simulink model "Demo_V2X_RoadWorks_cs"  (R2014b)
settings: Solver=ode5  SolverMode=SingleTasking  StartTime=0.0  StopTime=18  FixedStep=1/100  RelTol=1e-3
PreLoadFcn:
  | mbxruntime.callbacks.PreLoadFcn(bdroot);
  | check_NUTS_defined;
  | 
  | assignin('base',['model_closed_' bdroot],false);
PostLoadFcn:
  | mbxruntime.callbacks.PostLoadFcn(bdroot);
InitFcn:
  | mbxruntime.callbacks.InitFcn(bdroot);
StartFcn:
  | mbxruntime.callbacks.StartFcn(bdroot);
StopFcn:
  | mbxruntime.callbacks.StopFcn(bdroot);
model workspace: external: MAT-File .\Demo_V2X_RoadWorks_cs_hws.mat (data not in the file)
undefined symbols (not defined in the file or in its folder): InitializeBus, mbxruntime, Newton, Raphson, tabledata
undefined symbols (not defined in the file): Demo_V2X_RoadWorks_cs_002408181c311178, Demo_V2X_RoadWorks_cs_02afd40c5576fd79, Demo_V2X_RoadWorks_cs_09062d95c4976b80, Demo_V2X_RoadWorks_cs_0ad60e46608f1bfe, Demo_V2X_RoadWorks_cs_0b386a01b2cd5e8d, Demo_V2X_RoadWorks_cs_0d795afaa024d2ee, Demo_V2X_RoadWorks_cs_104085e65c337077, Demo_V2X_RoadWorks_cs_126564f7b2997a49, Demo_V2X_RoadWorks_cs_15e6e2595e8bf329, Demo_V2X_RoadWorks_cs_16adfea7655bce18, Demo_V2X_RoadWorks_cs_18ab2686f8449f50, Demo_V2X_RoadWorks_cs_1c28437def32f9f6, Demo_V2X_RoadWorks_cs_1d541c73c3d8f25b, Demo_V2X_RoadWorks_cs_1fb1f994fe012d27, Demo_V2X_RoadWorks_cs_20c117b9827230b9, Demo_V2X_RoadWorks_cs_220b1226a84e3b37, Demo_V2X_RoadWorks_cs_24814049c8ab2e18, Demo_V2X_RoadWorks_cs_24a281220a6492a7, Demo_V2X_RoadWorks_cs_279aea126b4236ad, Demo_V2X_RoadWorks_cs_28eadd0b23e572db, Demo_V2X_RoadWorks_cs_291fe7210f9ba434, Demo_V2X_RoadWorks_cs_2fd90504f8814746, Demo_V2X_RoadWorks_cs_33c1737bfc1c651f, Demo_V2X_RoadWorks_cs_388e22d5b1056b8f, Demo_V2X_RoadWorks_cs_3e3a415e868663e7, Demo_V2X_RoadWorks_cs_45759eb0c1816b1e, Demo_V2X_RoadWorks_cs_45f301cf6c396570, Demo_V2X_RoadWorks_cs_47686124f5151dea, Demo_V2X_RoadWorks_cs_487931e8a8cef1d6, Demo_V2X_RoadWorks_cs_54cb5626dca53ab7, Demo_V2X_RoadWorks_cs_56c0a253fe7e7ec0, Demo_V2X_RoadWorks_cs_5921488c0ba4168e, Demo_V2X_RoadWorks_cs_5ca0c70551eea1b3, Demo_V2X_RoadWorks_cs_5cc6ddb60eb17926, Demo_V2X_RoadWorks_cs_5dda33a127b53dd9, Demo_V2X_RoadWorks_cs_60729aca19e3b8ea, Demo_V2X_RoadWorks_cs_61616eaaf58ec115, Demo_V2X_RoadWorks_cs_63af626c9fae5224, Demo_V2X_RoadWorks_cs_649c6af7b111a61f, Demo_V2X_RoadWorks_cs_64e2df335ac415c1, Demo_V2X_RoadWorks_cs_6530f1ae727e39fe, Demo_V2X_RoadWorks_cs_6837be8d052ff1e3, Demo_V2X_RoadWorks_cs_6e8b51a123f1a201, Demo_V2X_RoadWorks_cs_6f4ec518a68cacb3, Demo_V2X_RoadWorks_cs_74dac4a6b9859226, Demo_V2X_RoadWorks_cs_75671d8cae67d5b6, Demo_V2X_RoadWorks_cs_756d40a88ae84d39, Demo_V2X_RoadWorks_cs_77c7cbc4fa1cdaa5, Demo_V2X_RoadWorks_cs_7b9fbc44403bb8f3, Demo_V2X_RoadWorks_cs_7c118b74c8d14c00, Demo_V2X_RoadWorks_cs_7c4a172761f05beb, Demo_V2X_RoadWorks_cs_80b7a78efe24d5f1, Demo_V2X_RoadWorks_cs_82d65efce1f7c4ea, Demo_V2X_RoadWorks_cs_8be5dc2565229ce9, Demo_V2X_RoadWorks_cs_8dc36f0ab6cec640, Demo_V2X_RoadWorks_cs_91305dd1362bb00d, Demo_V2X_RoadWorks_cs_929c2ffed1faf33f, Demo_V2X_RoadWorks_cs_95615bcbc0d062f1, Demo_V2X_RoadWorks_cs_99a6391a40f894df, Demo_V2X_RoadWorks_cs_9caa19175765ea5d ... (+52)
libraries: PreScanSimulinkLibrary x34, simulink_extras x15, simulink x6
(part 6 of 16)

== system Demo_V2X_RoadWorks_cs/V2X_Tx6196_DENM_Transmitter ==
  V2X_Tx6196_DENM_Transmitter : Inport  Tag=inport/plugin/sfun_V2X_DENM_Transmitter  BusOutputAsStruct=on
  Actuator : S-Function  FunctionName=sfun_V2X_DENM_Transmitter  Parameters=sensorID, parentID, timestep  EnableBusSupport=off  mask(V2X DENM Transmitter Block){sensorID=6196, parentID=3534, timestep=1/100}
      mask prompts: sensorID "Transmitter ID"; parentID "Parent ID"; timestep "MATLAB timestep:"
      mask help: V2X Block transmitting a DENM message
      mask Display: image(imread('V2XT_grayscale.png'))
  wires:
  V2X_Tx6196_DENM_Transmitter/1 -> Actuator/1

== system Demo_V2X_RoadWorks_cs/V2X_Tx6197_CAM_Transmitter ==
  V2X_Tx6197_CAM_Transmitter : Inport  Tag=inport/plugin/sfun_V2X_CAM_Transmitter  BusOutputAsStruct=on
  Actuator : S-Function  FunctionName=sfun_V2X_CAM_Transmitter  Parameters=sensorID, parentID, timestep  EnableBusSupport=off  mask(V2X CAM Transmitter Block){sensorID=6197, parentID=3535, timestep=1/100}
      mask prompts: sensorID "Transmitter ID"; parentID "Parent ID"; timestep "MATLAB timestep:"
      mask help: V2X Block transmitting a CAM message
      mask Display: image(imread('V2XT_grayscale.png'))
  wires:
  V2X_Tx6197_CAM_Transmitter/1 -> Actuator/1

== system Demo_V2X_RoadWorks_cs/V2X_Tx6197_DENM_Transmitter ==
  V2X_Tx6197_DENM_Transmitter : Inport  Tag=inport/plugin/sfun_V2X_DENM_Transmitter  BusOutputAsStruct=on
  Actuator : S-Function  FunctionName=sfun_V2X_DENM_Transmitter  Parameters=sensorID, parentID, timestep  EnableBusSupport=off  mask(V2X DENM Transmitter Block){sensorID=6197, parentID=3535, timestep=1/100}
      mask prompts: sensorID "Transmitter ID"; parentID "Parent ID"; timestep "MATLAB timestep:"
      mask help: V2X Block transmitting a DENM message
      mask Display: image(imread('V2XT_grayscale.png'))
  wires:
  V2X_Tx6197_DENM_Transmitter/1 -> Actuator/1

== system Demo_V2X_RoadWorks_cs/V2X_Tx6198_CAM_Transmitter ==
  V2X_Tx6198_CAM_Transmitter : Inport  Tag=inport/plugin/sfun_V2X_CAM_Transmitter  BusOutputAsStruct=on
  Actuator : S-Function  FunctionName=sfun_V2X_CAM_Transmitter  Parameters=sensorID, parentID, timestep  EnableBusSupport=off  mask(V2X CAM Transmitter Block){sensorID=6198, parentID=3606, timestep=1/100}
      mask prompts: sensorID "Transmitter ID"; parentID "Parent ID"; timestep "MATLAB timestep:"
      mask help: V2X Block transmitting a CAM message
      mask Display: image(imread('V2XT_grayscale.png'))
  wires:
  V2X_Tx6198_CAM_Transmitter/1 -> Actuator/1

== system Demo_V2X_RoadWorks_cs/V2X_Tx6198_DENM_Transmitter ==
  V2X_Tx6198_DENM_Transmitter : Inport  Tag=inport/plugin/sfun_V2X_DENM_Transmitter  BusOutputAsStruct=on
  Actuator : S-Function  FunctionName=sfun_V2X_DENM_Transmitter  Parameters=sensorID, parentID, timestep  EnableBusSupport=off  mask(V2X DENM Transmitter Block){sensorID=6198, parentID=3606, timestep=1/100}
      mask prompts: sensorID "Transmitter ID"; parentID "Parent ID"; timestep "MATLAB timestep:"
      mask help: V2X Block transmitting a DENM message
      mask Display: image(imread('V2XT_grayscale.png'))
  wires:
  V2X_Tx6198_DENM_Transmitter/1 -> Actuator/1

== system Demo_V2X_RoadWorks_cs/V2X_Tx6199_CAM_Transmitter ==
  V2X_Tx6199_CAM_Transmitter : Inport  Tag=inport/plugin/sfun_V2X_CAM_Transmitter  BusOutputAsStruct=on
  Actuator : S-Function  FunctionName=sfun_V2X_CAM_Transmitter  Parameters=sensorID, parentID, timestep  EnableBusSupport=off  mask(V2X CAM Transmitter Block){sensorID=6199, parentID=3607, timestep=1/100}
      mask prompts: sensorID "Transmitter ID"; parentID "Parent ID"; timestep "MATLAB timestep:"
      mask help: V2X Block transmitting a CAM message
      mask Display: image(imread('V2XT_grayscale.png'))
  wires:
  V2X_Tx6199_CAM_Transmitter/1 -> Actuator/1

== system Demo_V2X_RoadWorks_cs/V2X_Tx6199_DENM_Transmitter ==
  V2X_Tx6199_DENM_Transmitter : Inport  Tag=inport/plugin/sfun_V2X_DENM_Transmitter  BusOutputAsStruct=on
  Actuator : S-Function  FunctionName=sfun_V2X_DENM_Transmitter  Parameters=sensorID, parentID, timestep  EnableBusSupport=off  mask(V2X DENM Transmitter Block){sensorID=6199, parentID=3607, timestep=1/100}
      mask prompts: sensorID "Transmitter ID"; parentID "Parent ID"; timestep "MATLAB timestep:"
      mask help: V2X Block transmitting a DENM message
      mask Display: image(imread('V2XT_grayscale.png'))
  wires:
  V2X_Tx6199_DENM_Transmitter/1 -> Actuator/1

== system Demo_V2X_RoadWorks_cs/V2X_Tx6200_CAM_Transmitter ==
  V2X_Tx6200_CAM_Transmitter : Inport  Tag=inport/plugin/sfun_V2X_CAM_Transmitter  BusOutputAsStruct=on
  Actuator : S-Function  FunctionName=sfun_V2X_CAM_Transmitter  Parameters=sensorID, parentID, timestep  EnableBusSupport=off  mask(V2X CAM Transmitter Block){sensorID=6200, parentID=3608, timestep=1/100}
      mask prompts: sensorID "Transmitter ID"; parentID "Parent ID"; timestep "MATLAB timestep:"
      mask help: V2X Block transmitting a CAM message
      mask Display: image(imread('V2XT_grayscale.png'))
  wires:
  V2X_Tx6200_CAM_Transmitter/1 -> Actuator/1

== system Demo_V2X_RoadWorks_cs/V2X_Tx6200_DENM_Transmitter ==
  V2X_Tx6200_DENM_Transmitter : Inport  Tag=inport/plugin/sfun_V2X_DENM_Transmitter  BusOutputAsStruct=on
  Actuator : S-Function  FunctionName=sfun_V2X_DENM_Transmitter  Parameters=sensorID, parentID, timestep  EnableBusSupport=off  mask(V2X DENM Transmitter Block){sensorID=6200, parentID=3608, timestep=1/100}
      mask prompts: sensorID "Transmitter ID"; parentID "Parent ID"; timestep "MATLAB timestep:"
      mask help: V2X Block transmitting a DENM message
      mask Display: image(imread('V2XT_grayscale.png'))
  wires:
  V2X_Tx6200_DENM_Transmitter/1 -> Actuator/1

== system Demo_V2X_RoadWorks_cs/V2X_Tx6201_CAM_Transmitter ==
  V2X_Tx6201_CAM_Transmitter : Inport  Tag=inport/plugin/sfun_V2X_CAM_Transmitter  BusOutputAsStruct=on
  Actuator : S-Function  FunctionName=sfun_V2X_CAM_Transmitter  Parameters=sensorID, parentID, timestep  EnableBusSupport=off  mask(V2X CAM Transmitter Block){sensorID=6201, parentID=3609, timestep=1/100}
      mask prompts: sensorID "Transmitter ID"; parentID "Parent ID"; timestep "MATLAB timestep:"
      mask help: V2X Block transmitting a CAM message
      mask Display: image(imread('V2XT_grayscale.png'))
  wires:
  V2X_Tx6201_CAM_Transmitter/1 -> Actuator/1

== system Demo_V2X_RoadWorks_cs/V2X_Tx6201_DENM_Transmitter ==
  V2X_Tx6201_DENM_Transmitter : Inport  Tag=inport/plugin/sfun_V2X_DENM_Transmitter  BusOutputAsStruct=on
  Actuator : S-Function  FunctionName=sfun_V2X_DENM_Transmitter  Parameters=sensorID, parentID, timestep  EnableBusSupport=off  mask(V2X DENM Transmitter Block){sensorID=6201, parentID=3609, timestep=1/100}
      mask prompts: sensorID "Transmitter ID"; parentID "Parent ID"; timestep "MATLAB timestep:"
      mask help: V2X Block transmitting a DENM message
      mask Display: image(imread('V2XT_grayscale.png'))
  wires:
  V2X_Tx6201_DENM_Transmitter/1 -> Actuator/1

== system Demo_V2X_RoadWorks_cs/V2X_Tx6202_CAM_Transmitter ==
  V2X_Tx6202_CAM_Transmitter : Inport  Tag=inport/plugin/sfun_V2X_CAM_Transmitter  BusOutputAsStruct=on
  Actuator : S-Function  FunctionName=sfun_V2X_CAM_Transmitter  Parameters=sensorID, parentID, timestep  EnableBusSupport=off  mask(V2X CAM Transmitter Block){sensorID=6202, parentID=3711, timestep=1/100}
      mask prompts: sensorID "Transmitter ID"; parentID "Parent ID"; timestep "MATLAB timestep:"
      mask help: V2X Block transmitting a CAM message
      mask Display: image(imread('V2XT_grayscale.png'))
  wires:
  V2X_Tx6202_CAM_Transmitter/1 -> Actuator/1

== system Demo_V2X_RoadWorks_cs/V2X_Tx6202_DENM_Transmitter ==
  V2X_Tx6202_DENM_Transmitter : Inport  Tag=inport/plugin/sfun_V2X_DENM_Transmitter  BusOutputAsStruct=on
  Actuator : S-Function  FunctionName=sfun_V2X_DENM_Transmitter  Parameters=sensorID, parentID, timestep  EnableBusSupport=off  mask(V2X DENM Transmitter Block){sensorID=6202, parentID=3711, timestep=1/100}
      mask prompts: sensorID "Transmitter ID"; parentID "Parent ID"; timestep "MATLAB timestep:"
      mask help: V2X Block transmitting a DENM message
      mask Display: image(imread('V2XT_grayscale.png'))
  wires:
  V2X_Tx6202_DENM_Transmitter/1 -> Actuator/1

== system Demo_V2X_RoadWorks_cs/VISUColorRegion_Lower_Body_Male_Regular_BendingOver_1 ==
  VISUColorRegion_Lower_Body_Male_Regular_BendingOver_1 : Inport  Tag=inport/ColorRegion  OutDataTypeStr=Bus: PRESCAN_COLOR_DATA  PortDimensions=1  SampleTime=1/100  BusOutputAsStruct=on
  Actuator : S-Function  FunctionName=sfun_ColorActuator  Parameters=mbxruntime.parameters.convert(UniqueID), mbxruntime.parameters.convert(WorldModelSubPath),tabledata, TimeStep  EnableBusSupport=off  mask(PreScan Sink Block: VisuTextureColor){UniqueID=4029, WorldModelSubPath=/recolorRegion:name=Lower Body/targetColor, TimeStep=1/100}
      mask prompts: UniqueID "Parent Unique Identifier (auto-generated)"; WorldModelSubPath "WM SubPath(auto-generated)"; TimeStep "Simulink time step"
      mask help:
      | The VisuTextureColor block provides a way to adapt the color of a vehicle.
      |
      | For more information, please click Help.
      mask init:
      | [tabledata] = mbxruntime.parameters.table(UniqueID,WorldModelSubPath);
      mask Help: eval('openHelp(230)')
      mask Display: image(imread('TextureColor.png'))
  wires:
  VISUColorRegion_Lower_Body_Male_Regular_BendingOver_1/1 -> Actuator/1

== system Demo_V2X_RoadWorks_cs/VISUColorRegion_Lower_Body_Male_Regular_LeaningBack_1 ==
  VISUColorRegion_Lower_Body_Male_Regular_LeaningBack_1 : Inport  Tag=inport/ColorRegion  OutDataTypeStr=Bus: PRESCAN_COLOR_DATA  PortDimensions=1  SampleTime=1/100  BusOutputAsStruct=on
  Actuator : S-Function  FunctionName=sfun_ColorActuator  Parameters=mbxruntime.parameters.convert(UniqueID), mbxruntime.parameters.convert(WorldModelSubPath),tabledata, TimeStep  EnableBusSupport=off  mask(PreScan Sink Block: VisuTextureColor){UniqueID=4031, WorldModelSubPath=/recolorRegion:name=Lower Body/targetColor, TimeStep=1/100}
      mask prompts: UniqueID "Parent Unique Identifier (auto-generated)"; WorldModelSubPath "WM SubPath(auto-generated)"; TimeStep "Simulink time step"
      mask help:
      | The VisuTextureColor block provides a way to adapt the color of a vehicle.
      |
      | For more information, please click Help.
      mask init:
      | [tabledata] = mbxruntime.parameters.table(UniqueID,WorldModelSubPath);
      mask Help: eval('openHelp(230)')
      mask Display: image(imread('TextureColor.png'))
  wires:
  VISUColorRegion_Lower_Body_Male_Regular_LeaningBack_1/1 -> Actuator/1

== system Demo_V2X_RoadWorks_cs/VISUColorRegion_Lower_Body_Male_Regular_LeaningBack_2 ==
  VISUColorRegion_Lower_Body_Male_Regular_LeaningBack_2 : Inport  Tag=inport/ColorRegion  OutDataTypeStr=Bus: PRESCAN_COLOR_DATA  PortDimensions=1  SampleTime=1/100  BusOutputAsStruct=on
  Actuator : S-Function  FunctionName=sfun_ColorActuator  Parameters=mbxruntime.parameters.convert(UniqueID), mbxruntime.parameters.convert(WorldModelSubPath),tabledata, TimeStep  EnableBusSupport=off  mask(PreScan Sink Block: VisuTextureColor){UniqueID=4032, WorldModelSubPath=/recolorRegion:name=Lower Body/targetColor, TimeStep=1/100}
      mask prompts: UniqueID "Parent Unique Identifier (auto-generated)"; WorldModelSubPath "WM SubPath(auto-generated)"; TimeStep "Simulink time step"
      mask help:
      | The VisuTextureColor block provides a way to adapt the color of a vehicle.
      |
      | For more information, please click Help.
      mask init:
      | [tabledata] = mbxruntime.parameters.table(UniqueID,WorldModelSubPath);
      mask Help: eval('openHelp(230)')
      mask Display: image(imread('TextureColor.png'))
  wires:
  VISUColorRegion_Lower_Body_Male_Regular_LeaningBack_2/1 -> Actuator/1

== system Demo_V2X_RoadWorks_cs/VISUColorRegion_Lower_Body_Male_Regular_Leaning_1 ==
  VISUColorRegion_Lower_Body_Male_Regular_Leaning_1 : Inport  Tag=inport/ColorRegion  OutDataTypeStr=Bus: PRESCAN_COLOR_DATA  PortDimensions=1  SampleTime=1/100  BusOutputAsStruct=on
  Actuator : S-Function  FunctionName=sfun_ColorActuator  Parameters=mbxruntime.parameters.convert(UniqueID), mbxruntime.parameters.convert(WorldModelSubPath),tabledata, TimeStep  EnableBusSupport=off  mask(PreScan Sink Block: VisuTextureColor){UniqueID=4030, WorldModelSubPath=/recolorRegion:name=Lower Body/targetColor, TimeStep=1/100}
      mask prompts: UniqueID "Parent Unique Identifier (auto-generated)"; WorldModelSubPath "WM SubPath(auto-generated)"; TimeStep "Simulink time step"
      mask help:
      | The VisuTextureColor block provides a way to adapt the color of a vehicle.
      |
      | For more information, please click Help.
      mask init:
      | [tabledata] = mbxruntime.parameters.table(UniqueID,WorldModelSubPath);
      mask Help: eval('openHelp(230)')
      mask Display: image(imread('TextureColor.png'))
  wires:
  VISUColorRegion_Lower_Body_Male_Regular_Leaning_1/1 -> Actuator/1

== system Demo_V2X_RoadWorks_cs/VISUColorRegion_Lower_Body_Male_Regular_LyingDown_1 ==
  VISUColorRegion_Lower_Body_Male_Regular_LyingDown_1 : Inport  Tag=inport/ColorRegion  OutDataTypeStr=Bus: PRESCAN_COLOR_DATA  PortDimensions=1  SampleTime=1/100  BusOutputAsStruct=on
  Actuator : S-Function  FunctionName=sfun_ColorActuator  Parameters=mbxruntime.parameters.convert(UniqueID), mbxruntime.parameters.convert(WorldModelSubPath),tabledata, TimeStep  EnableBusSupport=off  mask(PreScan Sink Block: VisuTextureColor){UniqueID=4028, WorldModelSubPath=/recolorRegion:name=Lower Body/targetColor, TimeStep=1/100}
      mask prompts: UniqueID "Parent Unique Identifier (auto-generated)"; WorldModelSubPath "WM SubPath(auto-generated)"; TimeStep "Simulink time step"
      mask help:
      | The VisuTextureColor block provides a way to adapt the color of a vehicle.
      |
      | For more information, please click Help.
      mask init:
      | [tabledata] = mbxruntime.parameters.table(UniqueID,WorldModelSubPath);
      mask Help: eval('openHelp(230)')
      mask Display: image(imread('TextureColor.png'))
  wires:
  VISUColorRegion_Lower_Body_Male_Regular_LyingDown_1/1 -> Actuator/1

== system Demo_V2X_RoadWorks_cs/VISUColorRegion_Shoes_Male_Regular_BendingOver_1 ==
  VISUColorRegion_Shoes_Male_Regular_BendingOver_1 : Inport  Tag=inport/ColorRegion  OutDataTypeStr=Bus: PRESCAN_COLOR_DATA  PortDimensions=1  SampleTime=1/100  BusOutputAsStruct=on
  Actuator : S-Function  FunctionName=sfun_ColorActuator  Parameters=mbxruntime.parameters.convert(UniqueID), mbxruntime.parameters.convert(WorldModelSubPath),tabledata, TimeStep  EnableBusSupport=off  mask(PreScan Sink Block: VisuTextureColor){UniqueID=4029, WorldModelSubPath=/recolorRegion:name=Shoes/targetColor, TimeStep=1/100}
      mask prompts: UniqueID "Parent Unique Identifier (auto-generated)"; WorldModelSubPath "WM SubPath(auto-generated)"; TimeStep "Simulink time step"
      mask help:
      | The VisuTextureColor block provides a way to adapt the color of a vehicle.
      |
      | For more information, please click Help.
      mask init:
      | [tabledata] = mbxruntime.parameters.table(UniqueID,WorldModelSubPath);
      mask Help: eval('openHelp(230)')
      mask Display: image(imread('TextureColor.png'))
  wires:
  VISUColorRegion_Shoes_Male_Regular_BendingOver_1/1 -> Actuator/1

== system Demo_V2X_RoadWorks_cs/VISUColorRegion_Shoes_Male_Regular_LeaningBack_1 ==
  VISUColorRegion_Shoes_Male_Regular_LeaningBack_1 : Inport  Tag=inport/ColorRegion  OutDataTypeStr=Bus: PRESCAN_COLOR_DATA  PortDimensions=1  SampleTime=1/100  BusOutputAsStruct=on
  Actuator : S-Function  FunctionName=sfun_ColorActuator  Parameters=mbxruntime.parameters.convert(UniqueID), mbxruntime.parameters.convert(WorldModelSubPath),tabledata, TimeStep  EnableBusSupport=off  mask(PreScan Sink Block: VisuTextureColor){UniqueID=4031, WorldModelSubPath=/recolorRegion:name=Shoes/targetColor, TimeStep=1/100}
      mask prompts: UniqueID "Parent Unique Identifier (auto-generated)"; WorldModelSubPath "WM SubPath(auto-generated)"; TimeStep "Simulink time step"
      mask help:
      | The VisuTextureColor block provides a way to adapt the color of a vehicle.
      |
      | For more information, please click Help.
      mask init:
      | [tabledata] = mbxruntime.parameters.table(UniqueID,WorldModelSubPath);
      mask Help: eval('openHelp(230)')
      mask Display: image(imread('TextureColor.png'))
  wires:
  VISUColorRegion_Shoes_Male_Regular_LeaningBack_1/1 -> Actuator/1

== system Demo_V2X_RoadWorks_cs/VISUColorRegion_Shoes_Male_Regular_LeaningBack_2 ==
  VISUColorRegion_Shoes_Male_Regular_LeaningBack_2 : Inport  Tag=inport/ColorRegion  OutDataTypeStr=Bus: PRESCAN_COLOR_DATA  PortDimensions=1  SampleTime=1/100  BusOutputAsStruct=on
  Actuator : S-Function  FunctionName=sfun_ColorActuator  Parameters=mbxruntime.parameters.convert(UniqueID), mbxruntime.parameters.convert(WorldModelSubPath),tabledata, TimeStep  EnableBusSupport=off  mask(PreScan Sink Block: VisuTextureColor){UniqueID=4032, WorldModelSubPath=/recolorRegion:name=Shoes/targetColor, TimeStep=1/100}
      mask prompts: UniqueID "Parent Unique Identifier (auto-generated)"; WorldModelSubPath "WM SubPath(auto-generated)"; TimeStep "Simulink time step"
      mask help:
      | The VisuTextureColor block provides a way to adapt the color of a vehicle.
      |
      | For more information, please click Help.
      mask init:
      | [tabledata] = mbxruntime.parameters.table(UniqueID,WorldModelSubPath);
      mask Help: eval('openHelp(230)')
      mask Display: image(imread('TextureColor.png'))
  wires:
  VISUColorRegion_Shoes_Male_Regular_LeaningBack_2/1 -> Actuator/1

== system Demo_V2X_RoadWorks_cs/VISUColorRegion_Shoes_Male_Regular_Leaning_1 ==
  VISUColorRegion_Shoes_Male_Regular_Leaning_1 : Inport  Tag=inport/ColorRegion  OutDataTypeStr=Bus: PRESCAN_COLOR_DATA  PortDimensions=1  SampleTime=1/100  BusOutputAsStruct=on
  Actuator : S-Function  FunctionName=sfun_ColorActuator  Parameters=mbxruntime.parameters.convert(UniqueID), mbxruntime.parameters.convert(WorldModelSubPath),tabledata, TimeStep  EnableBusSupport=off  mask(PreScan Sink Block: VisuTextureColor){UniqueID=4030, WorldModelSubPath=/recolorRegion:name=Shoes/targetColor, TimeStep=1/100}
      mask prompts: UniqueID "Parent Unique Identifier (auto-generated)"; WorldModelSubPath "WM SubPath(auto-generated)"; TimeStep "Simulink time step"
      mask help:
      | The VisuTextureColor block provides a way to adapt the color of a vehicle.
      |
      | For more information, please click Help.
      mask init:
      | [tabledata] = mbxruntime.parameters.table(UniqueID,WorldModelSubPath);
      mask Help: eval('openHelp(230)')
      mask Display: image(imread('TextureColor.png'))
  wires:
  VISUColorRegion_Shoes_Male_Regular_Leaning_1/1 -> Actuator/1

== system Demo_V2X_RoadWorks_cs/VISUColorRegion_Shoes_Male_Regular_LyingDown_1 ==
  VISUColorRegion_Shoes_Male_Regular_LyingDown_1 : Inport  Tag=inport/ColorRegion  OutDataTypeStr=Bus: PRESCAN_COLOR_DATA  PortDimensions=1  SampleTime=1/100  BusOutputAsStruct=on
  Actuator : S-Function  FunctionName=sfun_ColorActuator  Parameters=mbxruntime.parameters.convert(UniqueID), mbxruntime.parameters.convert(WorldModelSubPath),tabledata, TimeStep  EnableBusSupport=off  mask(PreScan Sink Block: VisuTextureColor){UniqueID=4028, WorldModelSubPath=/recolorRegion:name=Shoes/targetColor, TimeStep=1/100}
      mask prompts: UniqueID "Parent Unique Identifier (auto-generated)"; WorldModelSubPath "WM SubPath(auto-generated)"; TimeStep "Simulink time step"
      mask help:
      | The VisuTextureColor block provides a way to adapt the color of a vehicle.
      |
      | For more information, please click Help.
      mask init:
      | [tabledata] = mbxruntime.parameters.table(UniqueID,WorldModelSubPath);
      mask Help: eval('openHelp(230)')
      mask Display: image(imread('TextureColor.png'))
  wires:
  VISUColorRegion_Shoes_Male_Regular_LyingDown_1/1 -> Actuator/1

== system Demo_V2X_RoadWorks_cs/VISUColorRegion_Upper_Body_Male_Regular_BendingOver_1 ==
  VISUColorRegion_Upper_Body_Male_Regular_BendingOver_1 : Inport  Tag=inport/ColorRegion  OutDataTypeStr=Bus: PRESCAN_COLOR_DATA  PortDimensions=1  SampleTime=1/100  BusOutputAsStruct=on
  Actuator : S-Function  FunctionName=sfun_ColorActuator  Parameters=mbxruntime.parameters.convert(UniqueID), mbxruntime.parameters.convert(WorldModelSubPath),tabledata, TimeStep  EnableBusSupport=off  mask(PreScan Sink Block: VisuTextureColor){UniqueID=4029, WorldModelSubPath=/recolorRegion:name=Upper Body/targetColor, TimeStep=1/100}
      mask prompts: UniqueID "Parent Unique Identifier (auto-generated)"; WorldModelSubPath "WM SubPath(auto-generated)"; TimeStep "Simulink time step"
      mask help:
      | The VisuTextureColor block provides a way to adapt the color of a vehicle.
      |
      | For more information, please click Help.
      mask init:
      | [tabledata] = mbxruntime.parameters.table(UniqueID,WorldModelSubPath);
      mask Help: eval('openHelp(230)')
      mask Display: image(imread('TextureColor.png'))
  wires:
  VISUColorRegion_Upper_Body_Male_Regular_BendingOver_1/1 -> Actuator/1

== system Demo_V2X_RoadWorks_cs/VISUColorRegion_Upper_Body_Male_Regular_LeaningBack_1 ==
  VISUColorRegion_Upper_Body_Male_Regular_LeaningBack_1 : Inport  Tag=inport/ColorRegion  OutDataTypeStr=Bus: PRESCAN_COLOR_DATA  PortDimensions=1  SampleTime=1/100  BusOutputAsStruct=on
  Actuator : S-Function  FunctionName=sfun_ColorActuator  Parameters=mbxruntime.parameters.convert(UniqueID), mbxruntime.parameters.convert(WorldModelSubPath),tabledata, TimeStep  EnableBusSupport=off  mask(PreScan Sink Block: VisuTextureColor){UniqueID=4031, WorldModelSubPath=/recolorRegion:name=Upper Body/targetColor, TimeStep=1/100}
      mask prompts: UniqueID "Parent Unique Identifier (auto-generated)"; WorldModelSubPath "WM SubPath(auto-generated)"; TimeStep "Simulink time step"
      mask help:
      | The VisuTextureColor block provides a way to adapt the color of a vehicle.
      |
      | For more information, please click Help.
      mask init:
      | [tabledata] = mbxruntime.parameters.table(UniqueID,WorldModelSubPath);
      mask Help: eval('openHelp(230)')
      mask Display: image(imread('TextureColor.png'))
  wires:
  VISUColorRegion_Upper_Body_Male_Regular_LeaningBack_1/1 -> Actuator/1

== system Demo_V2X_RoadWorks_cs/VISUColorRegion_Upper_Body_Male_Regular_LeaningBack_2 ==
  VISUColorRegion_Upper_Body_Male_Regular_LeaningBack_2 : Inport  Tag=inport/ColorRegion  OutDataTypeStr=Bus: PRESCAN_COLOR_DATA  PortDimensions=1  SampleTime=1/100  BusOutputAsStruct=on
  Actuator : S-Function  FunctionName=sfun_ColorActuator  Parameters=mbxruntime.parameters.convert(UniqueID), mbxruntime.parameters.convert(WorldModelSubPath),tabledata, TimeStep  EnableBusSupport=off  mask(PreScan Sink Block: VisuTextureColor){UniqueID=4032, WorldModelSubPath=/recolorRegion:name=Upper Body/targetColor, TimeStep=1/100}
      mask prompts: UniqueID "Parent Unique Identifier (auto-generated)"; WorldModelSubPath "WM SubPath(auto-generated)"; TimeStep "Simulink time step"
      mask help:
      | The VisuTextureColor block provides a way to adapt the color of a vehicle.
      |
      | For more information, please click Help.
      mask init:
      | [tabledata] = mbxruntime.parameters.table(UniqueID,WorldModelSubPath);
      mask Help: eval('openHelp(230)')
      mask Display: image(imread('TextureColor.png'))
  wires:
  VISUColorRegion_Upper_Body_Male_Regular_LeaningBack_2/1 -> Actuator/1

== system Demo_V2X_RoadWorks_cs/VISUColorRegion_Upper_Body_Male_Regular_Leaning_1 ==
  VISUColorRegion_Upper_Body_Male_Regular_Leaning_1 : Inport  Tag=inport/ColorRegion  OutDataTypeStr=Bus: PRESCAN_COLOR_DATA  PortDimensions=1  SampleTime=1/100  BusOutputAsStruct=on
  Actuator : S-Function  FunctionName=sfun_ColorActuator  Parameters=mbxruntime.parameters.convert(UniqueID), mbxruntime.parameters.convert(WorldModelSubPath),tabledata, TimeStep  EnableBusSupport=off  mask(PreScan Sink Block: VisuTextureColor){UniqueID=4030, WorldModelSubPath=/recolorRegion:name=Upper Body/targetColor, TimeStep=1/100}
      mask prompts: UniqueID "Parent Unique Identifier (auto-generated)"; WorldModelSubPath "WM SubPath(auto-generated)"; TimeStep "Simulink time step"
      mask help:
      | The VisuTextureColor block provides a way to adapt the color of a vehicle.
      |
      | For more information, please click Help.
      mask init:
      | [tabledata] = mbxruntime.parameters.table(UniqueID,WorldModelSubPath);
      mask Help: eval('openHelp(230)')
      mask Display: image(imread('TextureColor.png'))
  wires:
  VISUColorRegion_Upper_Body_Male_Regular_Leaning_1/1 -> Actuator/1

== system Demo_V2X_RoadWorks_cs/VISUColorRegion_Upper_Body_Male_Regular_LyingDown_1 ==
  VISUColorRegion_Upper_Body_Male_Regular_LyingDown_1 : Inport  Tag=inport/ColorRegion  OutDataTypeStr=Bus: PRESCAN_COLOR_DATA  PortDimensions=1  SampleTime=1/100  BusOutputAsStruct=on
  Actuator : S-Function  FunctionName=sfun_ColorActuator  Parameters=mbxruntime.parameters.convert(UniqueID), mbxruntime.parameters.convert(WorldModelSubPath),tabledata, TimeStep  EnableBusSupport=off  mask(PreScan Sink Block: VisuTextureColor){UniqueID=4028, WorldModelSubPath=/recolorRegion:name=Upper Body/targetColor, TimeStep=1/100}
      mask prompts: UniqueID "Parent Unique Identifier (auto-generated)"; WorldModelSubPath "WM SubPath(auto-generated)"; TimeStep "Simulink time step"
      mask help:
      | The VisuTextureColor block provides a way to adapt the color of a vehicle.
      |
      | For more information, please click Help.
      mask init:
      | [tabledata] = mbxruntime.parameters.table(UniqueID,WorldModelSubPath);
      mask Help: eval('openHelp(230)')
      mask Display: image(imread('TextureColor.png'))
  wires:
  VISUColorRegion_Upper_Body_Male_Regular_LyingDown_1/1 -> Actuator/1

== system Demo_V2X_RoadWorks_cs/WheelL0_Audi_A8_1 ==
  WheelL0_Audi_A8_1 : Inport  Tag=inport/JointActuator  OutDataTypeStr=Bus: PRESCAN_POSE_DATA  SampleTime=1/100  BusOutputAsStruct=on
  Actuator : Subsystem  Tag=VisuJoint  mask(PreScan Sink Block: VisuJoint){UniqueID=1227, Translate_ObjectID3D=Audi_A8_1.WheelL0, Rotate_ObjectID3D=Audi_A8_1.WheelL0, TimeStep=1/100, DisplayName=[]}
      mask prompts: UniqueID "Parent Unique ID"; Translate_ObjectID3D "Translate Object Name"; Rotate_ObjectID3D "Rotate Object Name"; TimeStep "Simulation Step"; DisplayName "Display Name"
      mask help:
      | The VisuJoint block provides a way to adapt the location and orientation of a part of an object.
      |
      | For more information, please click Help.
      settings: DeleteFcn=PreScanBlockDeleteFcn;
      mask Help: eval('openHelp(223)')
      mask Display: image(imread('Joint.png'))
  wires:
  WheelL0_Audi_A8_1/1 -> Actuator/1(Joint)

== system Demo_V2X_RoadWorks_cs/WheelL1_Audi_A8_1 ==
  WheelL1_Audi_A8_1 : Inport  Tag=inport/JointActuator  OutDataTypeStr=Bus: PRESCAN_POSE_DATA  SampleTime=1/100  BusOutputAsStruct=on
  Actuator : Subsystem  Tag=VisuJoint  mask(PreScan Sink Block: VisuJoint){UniqueID=1227, Translate_ObjectID3D=Audi_A8_1.WheelL1, Rotate_ObjectID3D=Audi_A8_1.WheelL1, TimeStep=1/100, DisplayName=[]}
      mask prompts: UniqueID "Parent Unique ID"; Translate_ObjectID3D "Translate Object Name"; Rotate_ObjectID3D "Rotate Object Name"; TimeStep "Simulation Step"; DisplayName "Display Name"
      mask help:
      | The VisuJoint block provides a way to adapt the location and orientation of a part of an object.
      |
      | For more information, please click Help.
      settings: DeleteFcn=PreScanBlockDeleteFcn;
      mask Help: eval('openHelp(223)')
      mask Display: image(imread('Joint.png'))
  wires:
  WheelL1_Audi_A8_1/1 -> Actuator/1(Joint)

== system Demo_V2X_RoadWorks_cs/WheelR0_Audi_A8_1 ==
  WheelR0_Audi_A8_1 : Inport  Tag=inport/JointActuator  OutDataTypeStr=Bus: PRESCAN_POSE_DATA  SampleTime=1/100  BusOutputAsStruct=on
  Actuator : Subsystem  Tag=VisuJoint  mask(PreScan Sink Block: VisuJoint){UniqueID=1227, Translate_ObjectID3D=Audi_A8_1.WheelR0, Rotate_ObjectID3D=Audi_A8_1.WheelR0, TimeStep=1/100, DisplayName=[]}
      mask prompts: UniqueID "Parent Unique ID"; Translate_ObjectID3D "Translate Object Name"; Rotate_ObjectID3D "Rotate Object Name"; TimeStep "Simulation Step"; DisplayName "Display Name"
      mask help:
      | The VisuJoint block provides a way to adapt the location and orientation of a part of an object.
      |
      | For more information, please click Help.
      settings: DeleteFcn=PreScanBlockDeleteFcn;
      mask Help: eval('openHelp(223)')
      mask Display: image(imread('Joint.png'))
  wires:
  WheelR0_Audi_A8_1/1 -> Actuator/1(Joint)

== system Demo_V2X_RoadWorks_cs/WheelR1_Audi_A8_1 ==
  WheelR1_Audi_A8_1 : Inport  Tag=inport/JointActuator  OutDataTypeStr=Bus: PRESCAN_POSE_DATA  SampleTime=1/100  BusOutputAsStruct=on
  Actuator : Subsystem  Tag=VisuJoint  mask(PreScan Sink Block: VisuJoint){UniqueID=1227, Translate_ObjectID3D=Audi_A8_1.WheelR1, Rotate_ObjectID3D=Audi_A8_1.WheelR1, TimeStep=1/100, DisplayName=[]}
      mask prompts: UniqueID "Parent Unique ID"; Translate_ObjectID3D "Translate Object Name"; Rotate_ObjectID3D "Rotate Object Name"; TimeStep "Simulation Step"; DisplayName "Display Name"
      mask help:
      | The VisuJoint block provides a way to adapt the location and orientation of a part of an object.
      |
      | For more information, please click Help.
      settings: DeleteFcn=PreScanBlockDeleteFcn;
      mask Help: eval('openHelp(223)')
      mask Display: image(imread('Joint.png'))
  wires:
  WheelR1_Audi_A8_1/1 -> Actuator/1(Joint)

== system Demo_V2X_RoadWorks_cs/Actros_1860_1/SELF_Demux ==
  SELF : Inport  OutDataTypeStr=Bus: PRESCAN_SELFSENSORDATA
  Bus Selector : BusSelector  OutputSignals=PositionX,PositionY,PositionZ,OrientationRoll,OrientationPitch,OrientationYaw,Velocity,Yaw_rate,Lat,Long,Alt
  Demux2 : Demux  Outputs=3
  Gain : Gain  Gain=180/pi
  Gain1 : Gain  Gain=180/pi
  Vector Concatenate1 : Concatenate  NumInputs=3
  compas converter : Subsystem
  x [m] : Outport
  y [m] : Outport  Port=2
  z [m] : Outport  Port=3
  rotx [deg] : Outport  Port=4
  roty [deg] : Outport  Port=5
  rotz [deg] : Outport  Port=6
  GPS lat [deg] : Outport  Port=7
  GPS long [deg] : Outport  Port=8
  GPS alt [m] : Outport  Port=9
  velocity [m/s] : Outport  Port=10
  heading [deg] : Outport  Port=11
  yaw rate [deg/s] : Outport  Port=12
  wires:
  Bus Selector/11 -> GPS alt [m]/1  "<Alt>"
  Bus Selector/10 -> GPS long [deg]/1  "<Long>"
  Bus Selector/9 -> GPS lat [deg]/1  "<Lat>"
  Bus Selector/8 -> Gain1/1  "<Yaw_rate>"
  Bus Selector/7 -> velocity [m/s]/1  "<Velocity>"
  Bus Selector/6 -> compas converter/1(rotz [rad]), Vector Concatenate1/3  "<OrientationYaw>"
  Bus Selector/5 -> Vector Concatenate1/2  "<OrientationPitch>"
  Bus Selector/4 -> Vector Concatenate1/1  "<OrientationRoll>"
  Vector Concatenate1/1 -> Gain/1
  Bus Selector/3 -> z [m]/1  "<PositionZ>"
  Bus Selector/2 -> y [m]/1  "<PositionY>"
  Bus Selector/1 -> x [m]/1  "<PositionX>"
  SELF/1 -> Bus Selector/1
  Gain/1 -> Demux2/1
  Demux2/1 -> rotx [deg]/1
  Demux2/2 -> roty [deg]/1
  Demux2/3 -> rotz [deg]/1
  compas converter/1(heading [deg]) -> heading [deg]/1
  Gain1/1 -> yaw rate [deg/s]/1

== system Demo_V2X_RoadWorks_cs/Actros_2541_1/Dynamics_Empty ==
  note: For state mode 'Dynamic' positions
      | are not taken into account, as they
      | are computed by integrating velocity.
      | Click annotation for Help.
  note: For state mode 'Dynamic' positions
      | are not taken into account, as they
      | are computed by integrating velocity.
      | Click annotation for Help.
  Ground_{1..9} (9 alike) : Ground
  MuxState : Subsystem  Tag=mux/State  mask(Empty Dynamics State Block){positioningmode=on, TimeStep=1/100}
      mask prompts: positioningmode "Positioning Mode"; TimeStep "Auto Assigned: Time Step [s]"
      mask help:
      | Build the state of an actor based on user input.
      | The user can either use positioning mode or dynamics mode.
      | - When using positioning mode the position and orientation of the actor are set directly based on the input. Expected input is relative to the initial position and orientation of the actor. It's also possible to specify the velocity of the actor, though this input isn't used, only passed on.
      | - When using dynamics mode the position input is ignored. Expected input is velocity and orientation. The velocity is relative the current orientation of the actor, while orientation is relative to its initial orientation. The position of the actor is calculated based on the velocity and orientation given.
      settings: DeleteFcn=PreScanBlockDeleteFcn;
  STATE_Actros_2541_1 : Subsystem  Tag=mux/StatePort  Priority=0  LoadFcn=load PrescanStateActuatorData  mask(PreScan Sink Block: State){x0=Demo_V2X_RoadWorks_cs_0d795afaa024d2ee, y0=Demo_V2X_RoadWorks_cs_c62d33b7dcd361f7, z0=Demo_V2X_RoadWorks_cs_15e6e2595e8bf329, Roll0=Demo_V2X_RoadWorks_cs_6f4ec518a68cacb3, Pitch0=Demo_V2X_RoadWorks_cs_7c118b74c8d14c00, Yaw0=Demo_V2X_RoadWorks_cs_64e2df335ac415c1, TimeStep=1/100}
      mask prompts: x0 "Ini x-position VEHICLE wrt GLOBAL axis system [m]"; y0 "Ini y-position VEHICLE wrt GLOBAL axis system [m]"; z0 "Ini z-position VEHICLE wrt GLOBAL axis system [m]"; Roll0 "Ini roll-angle BODY wrt VEHICLE axis system [deg]"; Pitch0 "Ini pitch-angle BODY wrt VEHICLE axis system [deg]"; Yaw0 "Ini yaw-angle VEHICLE wrt GLOBAL axis system [deg]"; TimeStep "Auto-Assigned: Upload Period [s]"
      mask help:
      | The Actor State contains a vector signal of size (9x1), containing the following signals:
      |
      | -  Position                  (x,y,z)                                     [m]
      | -  Velocity                  (vx,vy,vz)                               [m/s]
      | -  Angles                    (Roll, Pitch, Yaw)                   [rad]
      |
      | The Actor state is defined in the global axis system.
      | The state is superponed on the Initial position defined in the GUI.
      |
      | For more information, please click Help.
      settings: DeleteFcn=PreScanBlockDeleteFcn;
      mask Help: eval('openHelp(222)')
      mask Display: image(imread('State.png'))
  State : Outport  Tag=outport/StateOutport  SampleTime=1/100
  wires:
  MuxState/1(state) -> STATE_Actros_2541_1/1(State)
  STATE_Actros_2541_1/1(StateBus) -> State/1
  Ground_1/1 -> MuxState/1(x [m])
  Ground_2/1 -> MuxState/2(y [m])
  Ground_3/1 -> MuxState/3(z [m])
  Ground_4/1 -> MuxState/4(dx [m/s])
  Ground_5/1 -> MuxState/5(dy [m/s])
  Ground_6/1 -> MuxState/6(dz [m/s])
  Ground_7/1 -> MuxState/7(R [rad])
  Ground_8/1 -> MuxState/8(P [rad])
  Ground_9/1 -> MuxState/9(Y [rad])

== system Demo_V2X_RoadWorks_cs/Actros_2541_1/SELF_Demux ==
  SELF : Inport  OutDataTypeStr=Bus: PRESCAN_SELFSENSORDATA
  Bus Selector : BusSelector  OutputSignals=PositionX,PositionY,PositionZ,OrientationRoll,OrientationPitch,OrientationYaw,Velocity,Yaw_rate,Lat,Long,Alt
  Demux2 : Demux  Outputs=3
  Gain : Gain  Gain=180/pi
  Gain1 : Gain  Gain=180/pi
  Vector Concatenate1 : Concatenate  NumInputs=3
  compas converter : Subsystem
  x [m] : Outport
  y [m] : Outport  Port=2
  z [m] : Outport  Port=3
  rotx [deg] : Outport  Port=4
  roty [deg] : Outport  Port=5
  rotz [deg] : Outport  Port=6
  GPS lat [deg] : Outport  Port=7
  GPS long [deg] : Outport  Port=8
  GPS alt [m] : Outport  Port=9
  velocity [m/s] : Outport  Port=10
  heading [deg] : Outport  Port=11
  yaw rate [deg/s] : Outport  Port=12
  wires:
  Bus Selector/11 -> GPS alt [m]/1  "<Alt>"
  Bus Selector/10 -> GPS long [deg]/1  "<Long>"
  Bus Selector/9 -> GPS lat [deg]/1  "<Lat>"
  Bus Selector/8 -> Gain1/1  "<Yaw_rate>"
  Bus Selector/7 -> velocity [m/s]/1  "<Velocity>"
  Bus Selector/6 -> compas converter/1(rotz [rad]), Vector Concatenate1/3  "<OrientationYaw>"
  Bus Selector/5 -> Vector Concatenate1/2  "<OrientationPitch>"
  Bus Selector/4 -> Vector Concatenate1/1  "<OrientationRoll>"
  Vector Concatenate1/1 -> Gain/1
  Bus Selector/3 -> z [m]/1  "<PositionZ>"
  Bus Selector/2 -> y [m]/1  "<PositionY>"
  Bus Selector/1 -> x [m]/1  "<PositionX>"
  SELF/1 -> Bus Selector/1
  Gain/1 -> Demux2/1
  Demux2/1 -> rotx [deg]/1
  Demux2/2 -> roty [deg]/1
  Demux2/3 -> rotz [deg]/1
  compas converter/1(heading [deg]) -> heading [deg]/1
  Gain1/1 -> yaw rate [deg/s]/1

== system Demo_V2X_RoadWorks_cs/Audi_A8_1/Brake_light_left_Mux ==
  MSCD [Cd] : Inport
  Position (xyz) [m] : Inport  Port=2
  Orientation (RPY) [deg] : Inport  Port=3
  Color [-] : Inport  Port=4
  TextureResourceID [-] : Inport  Port=5
  Bus Creator : BusCreator  Inputs='Intensity','Position','Orientation','Color','TextureResourceID'  OutDataTypeStr=Bus: PRESCAN_VISULIGHTACTUATOR_DATA  NonVirtualBus=on
  Bus Creator1 : BusCreator  Inputs=3  OutDataTypeStr=Bus: PRESCAN_RGB_DATA  NonVirtualBus=on
  Bus Creator2 : BusCreator  Inputs=3  OutDataTypeStr=Bus: PRESCAN_RPY_DATA  NonVirtualBus=on
  Bus Creator3 : BusCreator  Inputs=3  OutDataTypeStr=Bus: PRESCAN_XYZ_DATA  NonVirtualBus=on
  Data Type Conversion : DataTypeConversion  OutDataTypeStr=int32  RndMeth=Nearest
  Degrees to Radians : simulink_extras/Transformations/Degrees to Radians
  Demux : Demux  Outputs=3
  Demux1 : Demux  Outputs=3
  Demux2 : Demux  Outputs=3
  Lights : Outport
  wires:
  TextureResourceID [-]/1 -> Data Type Conversion/1  "TextureResourceID"
  MSCD [Cd]/1 -> Bus Creator/1  "Intensity"
  Bus Creator/1 -> Lights/1
  Demux/1 -> Bus Creator1/1  "R"
  Demux/2 -> Bus Creator1/2  "G"
  Demux/3 -> Bus Creator1/3  "B"
  Color [-]/1 -> Demux/1  "Color"
  Bus Creator1/1 -> Bus Creator/4  "Color"
  Demux1/1 -> Bus Creator2/1  "Roll"
  Demux1/2 -> Bus Creator2/2  "Pitch"
  Demux1/3 -> Bus Creator2/3  "Yaw"
  Orientation (RPY) [deg]/1 -> Degrees to Radians/1  "Orientation"
  Bus Creator2/1 -> Bus Creator/3  "Orientation"
  Demux2/1 -> Bus Creator3/1  "X"
  Demux2/2 -> Bus Creator3/2  "Y"
  Demux2/3 -> Bus Creator3/3  "Z"
  Position (xyz) [m]/1 -> Demux2/1  "Position"
  Bus Creator3/1 -> Bus Creator/2  "Position"
  Data Type Conversion/1 -> Bus Creator/5  "TextureResourceID"
  Degrees to Radians/1 -> Demux1/1

== system Demo_V2X_RoadWorks_cs/Audi_A8_1/Brake_light_right_Mux ==
  MSCD [Cd] : Inport
  Position (xyz) [m] : Inport  Port=2
  Orientation (RPY) [deg] : Inport  Port=3
  Color [-] : Inport  Port=4
  TextureResourceID [-] : Inport  Port=5
  Bus Creator : BusCreator  Inputs='Intensity','Position','Orientation','Color','TextureResourceID'  OutDataTypeStr=Bus: PRESCAN_VISULIGHTACTUATOR_DATA  NonVirtualBus=on
  Bus Creator1 : BusCreator  Inputs=3  OutDataTypeStr=Bus: PRESCAN_RGB_DATA  NonVirtualBus=on
  Bus Creator2 : BusCreator  Inputs=3  OutDataTypeStr=Bus: PRESCAN_RPY_DATA  NonVirtualBus=on
  Bus Creator3 : BusCreator  Inputs=3  OutDataTypeStr=Bus: PRESCAN_XYZ_DATA  NonVirtualBus=on
  Data Type Conversion : DataTypeConversion  OutDataTypeStr=int32  RndMeth=Nearest
  Degrees to Radians : simulink_extras/Transformations/Degrees to Radians
  Demux : Demux  Outputs=3
  Demux1 : Demux  Outputs=3
  Demux2 : Demux  Outputs=3
  Lights : Outport
  wires:
  TextureResourceID [-]/1 -> Data Type Conversion/1  "TextureResourceID"
  MSCD [Cd]/1 -> Bus Creator/1  "Intensity"
  Bus Creator/1 -> Lights/1
  Demux/1 -> Bus Creator1/1  "R"
  Demux/2 -> Bus Creator1/2  "G"
  Demux/3 -> Bus Creator1/3  "B"
  Color [-]/1 -> Demux/1  "Color"
  Bus Creator1/1 -> Bus Creator/4  "Color"
  Demux1/1 -> Bus Creator2/1  "Roll"
  Demux1/2 -> Bus Creator2/2  "Pitch"
  Demux1/3 -> Bus Creator2/3  "Yaw"
  Orientation (RPY) [deg]/1 -> Degrees to Radians/1  "Orientation"
  Bus Creator2/1 -> Bus Creator/3  "Orientation"
  Demux2/1 -> Bus Creator3/1  "X"
  Demux2/2 -> Bus Creator3/2  "Y"
  Demux2/3 -> Bus Creator3/3  "Z"
  Position (xyz) [m]/1 -> Demux2/1  "Position"
  Bus Creator3/1 -> Bus Creator/2  "Position"
  Data Type Conversion/1 -> Bus Creator/5  "TextureResourceID"
  Degrees to Radians/1 -> Demux1/1

== system Demo_V2X_RoadWorks_cs/Audi_A8_1/Braking ==
  V : Inport
  Compare To Constant : simulink/Logic and Bit Operations/Compare To Constant  relop=<  const=-1e-6  OutDataTypeStr=boolean
  Data Type Conversion : DataTypeConversion  OutDataTypeStr=double
  Difference : simulink/Discrete/Difference  ICPrevInput=0.0  InputProcessing=Inherited  OutMin=[]  OutMax=[]  OutDataType=fixdt(1, 16)  OutScaling=2^-10  DoSatur=off
  Scope : Scope
  Scope1 : Scope
      settings: SaveName=ScopeData10
  Scope2 : Scope
      settings: YMin=1  YMax=1  SaveName=ScopeData11
  B : Outport
  wires:
  V/1 -> Difference/1, Scope/1
  Difference/1 -> Scope1/1, Compare To Constant/1
  Data Type Conversion/1 -> B/1
  Compare To Constant/1 -> Data Type Conversion/1, Scope2/1

== system Demo_V2X_RoadWorks_cs/Audi_A8_1/Indicator_front_left_Mux ==
  MSCD [Cd] : Inport
  Position (xyz) [m] : Inport  Port=2
  Orientation (RPY) [deg] : Inport  Port=3
  Color [-] : Inport  Port=4
  TextureResourceID [-] : Inport  Port=5
  Bus Creator : BusCreator  Inputs='Intensity','Position','Orientation','Color','TextureResourceID'  OutDataTypeStr=Bus: PRESCAN_VISULIGHTACTUATOR_DATA  NonVirtualBus=on
  Bus Creator1 : BusCreator  Inputs=3  OutDataTypeStr=Bus: PRESCAN_RGB_DATA  NonVirtualBus=on
  Bus Creator2 : BusCreator  Inputs=3  OutDataTypeStr=Bus: PRESCAN_RPY_DATA  NonVirtualBus=on
  Bus Creator3 : BusCreator  Inputs=3  OutDataTypeStr=Bus: PRESCAN_XYZ_DATA  NonVirtualBus=on
  Data Type Conversion : DataTypeConversion  OutDataTypeStr=int32  RndMeth=Nearest
  Degrees to Radians : simulink_extras/Transformations/Degrees to Radians
  Demux : Demux  Outputs=3
  Demux1 : Demux  Outputs=3
  Demux2 : Demux  Outputs=3
  Lights : Outport
  wires:
  TextureResourceID [-]/1 -> Data Type Conversion/1  "TextureResourceID"
  MSCD [Cd]/1 -> Bus Creator/1  "Intensity"
  Bus Creator/1 -> Lights/1
  Demux/1 -> Bus Creator1/1  "R"
  Demux/2 -> Bus Creator1/2  "G"
  Demux/3 -> Bus Creator1/3  "B"
  Color [-]/1 -> Demux/1  "Color"
  Bus Creator1/1 -> Bus Creator/4  "Color"
  Demux1/1 -> Bus Creator2/1  "Roll"
  Demux1/2 -> Bus Creator2/2  "Pitch"
  Demux1/3 -> Bus Creator2/3  "Yaw"
  Orientation (RPY) [deg]/1 -> Degrees to Radians/1  "Orientation"
  Bus Creator2/1 -> Bus Creator/3  "Orientation"
  Demux2/1 -> Bus Creator3/1  "X"
  Demux2/2 -> Bus Creator3/2  "Y"
  Demux2/3 -> Bus Creator3/3  "Z"
  Position (xyz) [m]/1 -> Demux2/1  "Position"
  Bus Creator3/1 -> Bus Creator/2  "Position"
  Data Type Conversion/1 -> Bus Creator/5  "TextureResourceID"
  Degrees to Radians/1 -> Demux1/1

== system Demo_V2X_RoadWorks_cs/Audi_A8_1/Indicator_front_right_Mux ==
  MSCD [Cd] : Inport
  Position (xyz) [m] : Inport  Port=2
  Orientation (RPY) [deg] : Inport  Port=3
  Color [-] : Inport  Port=4
  TextureResourceID [-] : Inport  Port=5
  Bus Creator : BusCreator  Inputs='Intensity','Position','Orientation','Color','TextureResourceID'  OutDataTypeStr=Bus: PRESCAN_VISULIGHTACTUATOR_DATA  NonVirtualBus=on
  Bus Creator1 : BusCreator  Inputs=3  OutDataTypeStr=Bus: PRESCAN_RGB_DATA  NonVirtualBus=on
  Bus Creator2 : BusCreator  Inputs=3  OutDataTypeStr=Bus: PRESCAN_RPY_DATA  NonVirtualBus=on
  Bus Creator3 : BusCreator  Inputs=3  OutDataTypeStr=Bus: PRESCAN_XYZ_DATA  NonVirtualBus=on
  Data Type Conversion : DataTypeConversion  OutDataTypeStr=int32  RndMeth=Nearest
  Degrees to Radians : simulink_extras/Transformations/Degrees to Radians
  Demux : Demux  Outputs=3
  Demux1 : Demux  Outputs=3
  Demux2 : Demux  Outputs=3
  Lights : Outport
  wires:
  TextureResourceID [-]/1 -> Data Type Conversion/1  "TextureResourceID"
  MSCD [Cd]/1 -> Bus Creator/1  "Intensity"
  Bus Creator/1 -> Lights/1
  Demux/1 -> Bus Creator1/1  "R"
  Demux/2 -> Bus Creator1/2  "G"
  Demux/3 -> Bus Creator1/3  "B"
  Color [-]/1 -> Demux/1  "Color"
  Bus Creator1/1 -> Bus Creator/4  "Color"
  Demux1/1 -> Bus Creator2/1  "Roll"
  Demux1/2 -> Bus Creator2/2  "Pitch"
  Demux1/3 -> Bus Creator2/3  "Yaw"
  Orientation (RPY) [deg]/1 -> Degrees to Radians/1  "Orientation"
  Bus Creator2/1 -> Bus Creator/3  "Orientation"
  Demux2/1 -> Bus Creator3/1  "X"
  Demux2/2 -> Bus Creator3/2  "Y"
  Demux2/3 -> Bus Creator3/3  "Z"
  Position (xyz) [m]/1 -> Demux2/1  "Position"
  Bus Creator3/1 -> Bus Creator/2  "Position"
  Data Type Conversion/1 -> Bus Creator/5  "TextureResourceID"
  Degrees to Radians/1 -> Demux1/1

== system Demo_V2X_RoadWorks_cs/Audi_A8_1/Indicator_rear_left_Mux ==
  MSCD [Cd] : Inport
  Position (xyz) [m] : Inport  Port=2
  Orientation (RPY) [deg] : Inport  Port=3
  Color [-] : Inport  Port=4
  TextureResourceID [-] : Inport  Port=5
  Bus Creator : BusCreator  Inputs='Intensity','Position','Orientation','Color','TextureResourceID'  OutDataTypeStr=Bus: PRESCAN_VISULIGHTACTUATOR_DATA  NonVirtualBus=on
  Bus Creator1 : BusCreator  Inputs=3  OutDataTypeStr=Bus: PRESCAN_RGB_DATA  NonVirtualBus=on
  Bus Creator2 : BusCreator  Inputs=3  OutDataTypeStr=Bus: PRESCAN_RPY_DATA  NonVirtualBus=on
  Bus Creator3 : BusCreator  Inputs=3  OutDataTypeStr=Bus: PRESCAN_XYZ_DATA  NonVirtualBus=on
  Data Type Conversion : DataTypeConversion  OutDataTypeStr=int32  RndMeth=Nearest
  Degrees to Radians : simulink_extras/Transformations/Degrees to Radians
  Demux : Demux  Outputs=3
  Demux1 : Demux  Outputs=3
  Demux2 : Demux  Outputs=3
  Lights : Outport
  wires:
  TextureResourceID [-]/1 -> Data Type Conversion/1  "TextureResourceID"
  MSCD [Cd]/1 -> Bus Creator/1  "Intensity"
  Bus Creator/1 -> Lights/1
  Demux/1 -> Bus Creator1/1  "R"
  Demux/2 -> Bus Creator1/2  "G"
  Demux/3 -> Bus Creator1/3  "B"
  Color [-]/1 -> Demux/1  "Color"
  Bus Creator1/1 -> Bus Creator/4  "Color"
  Demux1/1 -> Bus Creator2/1  "Roll"
  Demux1/2 -> Bus Creator2/2  "Pitch"
  Demux1/3 -> Bus Creator2/3  "Yaw"
  Orientation (RPY) [deg]/1 -> Degrees to Radians/1  "Orientation"
  Bus Creator2/1 -> Bus Creator/3  "Orientation"
  Demux2/1 -> Bus Creator3/1  "X"
  Demux2/2 -> Bus Creator3/2  "Y"
  Demux2/3 -> Bus Creator3/3  "Z"
  Position (xyz) [m]/1 -> Demux2/1  "Position"
  Bus Creator3/1 -> Bus Creator/2  "Position"
  Data Type Conversion/1 -> Bus Creator/5  "TextureResourceID"
  Degrees to Radians/1 -> Demux1/1

== system Demo_V2X_RoadWorks_cs/Audi_A8_1/Indicator_rear_right_Mux ==
  MSCD [Cd] : Inport
  Position (xyz) [m] : Inport  Port=2
  Orientation (RPY) [deg] : Inport  Port=3
  Color [-] : Inport  Port=4
  TextureResourceID [-] : Inport  Port=5
  Bus Creator : BusCreator  Inputs='Intensity','Position','Orientation','Color','TextureResourceID'  OutDataTypeStr=Bus: PRESCAN_VISULIGHTACTUATOR_DATA  NonVirtualBus=on
  Bus Creator1 : BusCreator  Inputs=3  OutDataTypeStr=Bus: PRESCAN_RGB_DATA  NonVirtualBus=on
  Bus Creator2 : BusCreator  Inputs=3  OutDataTypeStr=Bus: PRESCAN_RPY_DATA  NonVirtualBus=on
  Bus Creator3 : BusCreator  Inputs=3  OutDataTypeStr=Bus: PRESCAN_XYZ_DATA  NonVirtualBus=on
  Data Type Conversion : DataTypeConversion  OutDataTypeStr=int32  RndMeth=Nearest
  Degrees to Radians : simulink_extras/Transformations/Degrees to Radians
  Demux : Demux  Outputs=3
  Demux1 : Demux  Outputs=3
  Demux2 : Demux  Outputs=3
  Lights : Outport
  wires:
  TextureResourceID [-]/1 -> Data Type Conversion/1  "TextureResourceID"
  MSCD [Cd]/1 -> Bus Creator/1  "Intensity"
  Bus Creator/1 -> Lights/1
  Demux/1 -> Bus Creator1/1  "R"
  Demux/2 -> Bus Creator1/2  "G"
  Demux/3 -> Bus Creator1/3  "B"
  Color [-]/1 -> Demux/1  "Color"
  Bus Creator1/1 -> Bus Creator/4  "Color"
  Demux1/1 -> Bus Creator2/1  "Roll"
  Demux1/2 -> Bus Creator2/2  "Pitch"
  Demux1/3 -> Bus Creator2/3  "Yaw"
  Orientation (RPY) [deg]/1 -> Degrees to Radians/1  "Orientation"
  Bus Creator2/1 -> Bus Creator/3  "Orientation"
  Demux2/1 -> Bus Creator3/1  "X"
  Demux2/2 -> Bus Creator3/2  "Y"
  Demux2/3 -> Bus Creator3/3  "Z"
  Position (xyz) [m]/1 -> Demux2/1  "Position"
  Bus Creator3/1 -> Bus Creator/2  "Position"
  Data Type Conversion/1 -> Bus Creator/5  "TextureResourceID"
  Degrees to Radians/1 -> Demux1/1

== system Demo_V2X_RoadWorks_cs/Audi_A8_1/JointGroup_WheelDisplacement_V2R ==
  Velocity [m/s] : Inport  SampleTime=TimeStep
  Discrete-Time Integrator : DiscreteIntegrator  SampleTime=TimeStep
  omega=V/Rwheel : Gain  Gain=1/TireRadius
  Rotation [rad] : Outport
  wires:
  Discrete-Time Integrator/1 -> Rotation [rad]/1  "roty"
  omega=V/Rwheel/1 -> Discrete-Time Integrator/1  "rotational speed [rad/s]"
  Velocity [m/s]/1 -> omega=V/Rwheel/1
